simulink model "Server"  (R2016a)
settings: Solver=VariableStepAuto  StartTime=0.0  StopTime=0  RelTol=1e-3
settings Model: Creator=Hilals  LastModifiedBy=Hilals

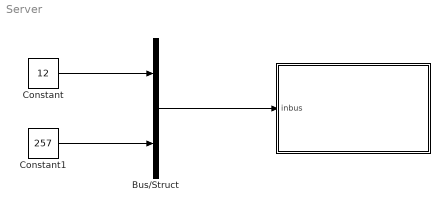
== system Server ==
  " " : MATLAB Function  TreatAsAtomicUnit=on  mask(TcpIpSendServer){IP=uint8('0.0.0.0'), Port=47806}
      mask prompts: IP "Remote IP Address"; Port "Remote Port"
      mask help: Send Data to Client Side
  Bus/Struct : BusCreator  Inputs=2  OutDataTypeStr=Bus: Bus  NonVirtualBus=on
  Constant : Constant  Value=12
  Constant1 : Constant  Value=257
  wires:
  Constant/1 -> Bus/Struct/1
  Constant1/1 -> Bus/Struct/2
  Bus/Struct/1 -> " "/1(inbus)

== matlab function Server/  ==
  data: inbus input Bus: Bus; IP parameter; Port parameter
function fcn(inbus, IP, Port)
coder.extrinsic('tcpip'); % codegen
coder.extrinsic('fwrite'); % codegen
coder.extrinsic('cell2mat'); % codegen

% Char is not supported by MATLAB. Input Parameter from Simulink is uint8!!
% for this reason;
ipAddress = char(IP);

%% struct --> cell array --> matrix
% 2016a MATLAB problem. If you have 2016b or latest version, 
% you could use json format to send struct data (bkz:jsonencode,jsondecode)
dataCell = struct2cell(inbus);
data = cell2mat(dataCell);

%% Tcp\IP
t = tcpip(ipAddress,Port,'NetworkRole','server');
fopen(t); % wait client

%% Connected
fwrite(t,data,'double');
